simulink model "RR_interaction"  (R2020b)
settings: Solver=FixedStepAuto  StartTime=0.0  StopTime=10.0  FixedStep=0.001  MaxStep=0.05  RelTol=1e-3
values from neighbouring files (symbols this model uses):
  e_max = 0.01    [init.m]
  F_int_max = [5;5]    [init.m]
  F_max = [4;4]    [init.m]
  g = 9.81    [init.m]
  I1 = 1    [init.m]
  I2 = 1    [init.m]
  l1 = 1    [init.m]
  l2 = 1    [init.m]
  m1 = 1    [init.m]
  m2 = 1    [init.m]
  mass = 1    [init.m]
  ts_bound = 0.05    [init.m]
libraries: cstblocks x2, simulink x1
settings Model: Creator=chiara-s  LastModifiedBy=chiara-s

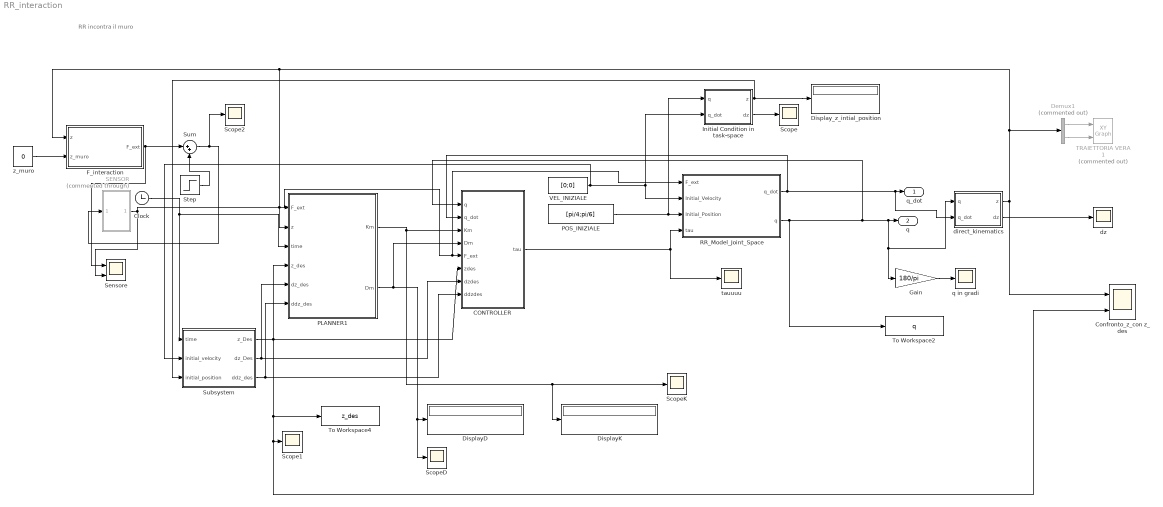
== system RR_interaction ==
  note: RR incontra il muro
  CONTROLLER : MATLAB Function  TreatAsAtomicUnit=on
  Clock : Clock
  Confronto_z_con z_des : Scope  NumInputPorts=2
  Demux1 : Demux  Commented=on  Outputs=2
  DisplayD : Display
  DisplayK : Display
  Display_z_intial_position : Display
  F_interaction : MATLAB Function  TreatAsAtomicUnit=on
  Gain : Gain  Gain=180/pi
  Initial Condition in task-space : MATLAB Function  TreatAsAtomicUnit=on
  PLANNER1 : MATLAB Function  TreatAsAtomicUnit=on
  POS_INIZIALE : Constant  Value=[pi/4;pi/6]
  RR_Model_Joint_Space : Subsystem
  SENSOR : Subsystem  Commented=through
  Scope : Scope
  Scope1 : Scope
  Scope2 : Scope
  ScopeD : Scope
  ScopeK : Scope
  "Sensore " : Scope  NumInputPorts=2
  Step : Step  Time=0  After=[F_max(1);0]  SampleTime=0
  Subsystem : Subsystem
  Sum : Sum  Inputs=|++
  TRAIETTORIA VERA 1 : simulink/Sinks/XY Graph  Commented=on  xmin=-2  xmax=2  ymin=-2  ymax=2  st=-1
  To Workspace2 : ToWorkspace  VariableName=q  SaveFormat=Structure With Time  SampleTime=-1
      settings: Save2DSignal=2-D array (concatenate along first dimension)
  To Workspace4 : ToWorkspace  VariableName=z_des  SaveFormat=Structure With Time  SampleTime=-1
      settings: Save2DSignal=2-D array (concatenate along first dimension)
  VEL_INIZIALE : Constant  Value=[0;0]
  direct_kinematics : MATLAB Function  TreatAsAtomicUnit=on
  dz : Scope
  q in gradi : Scope
  tauuuu : Scope
  z_muro : Constant  Value=0
  q_dot : Outport
  q : Outport  Port=2
  wires:
  z_muro/1 -> F_interaction/2(z_muro)
  direct_kinematics/1(z) -> Confronto_z_con z_des/1, PLANNER1/2(z), F_interaction/1(z), Demux1/1
  Clock/1 -> Subsystem/1(time), PLANNER1/3(time)
  Demux1/2 -> TRAIETTORIA VERA 1/2
  Subsystem/2(dz_Des) -> PLANNER1/5(dz_des), CONTROLLER/7(dzdes)
  VEL_INIZIALE/1 -> Subsystem/2(initial_velocity), Initial Condition in task-space/2(q_dot), RR_Model_Joint_Space/2(Initial_Velocity)
  CONTROLLER/1(tau) -> tauuuu/1, RR_Model_Joint_Space/4(tau)
  Initial Condition in task-space/2(dz) -> Scope/1
  direct_kinematics/2(dz) -> dz/1
  Subsystem/1(z_Des) -> PLANNER1/4(z_des), CONTROLLER/6(zdes), Confronto_z_con z_des/2, Scope1/1, To Workspace4/1
  POS_INIZIALE/1 -> RR_Model_Joint_Space/3(Initial_Position), Initial Condition in task-space/1(q)
  RR_Model_Joint_Space/2(q) -> CONTROLLER/1(q), Gain/1, direct_kinematics/1(q), q/1, To Workspace2/1
  Subsystem/3(ddz_des) -> PLANNER1/6(ddz_des), CONTROLLER/8(ddzdes)
  SENSOR/1(F_ext) -> RR_Model_Joint_Space/1(F_ext), CONTROLLER/5(F_ext), PLANNER1/1(F_ext), "Sensore "/2
  Gain/1 -> q in gradi/1
  Initial Condition in task-space/1(z) -> Subsystem/3(initial_position), Display_z_intial_position/1
  RR_Model_Joint_Space/1(q_dot) -> direct_kinematics/2(q_dot), q_dot/1, CONTROLLER/2(q_dot)
  Demux1/1 -> TRAIETTORIA VERA 1/1
  PLANNER1/1(Km) -> DisplayK/1, ScopeK/1, CONTROLLER/3(Km)
  PLANNER1/2(Dm) -> CONTROLLER/4(Dm), ScopeD/1, DisplayD/1
  F_interaction/1(F_ext) -> "Sensore "/1, Sum/1
  Sum/1 -> Scope2/1, SENSOR/1(In1)
  Step/1 -> Sum/2

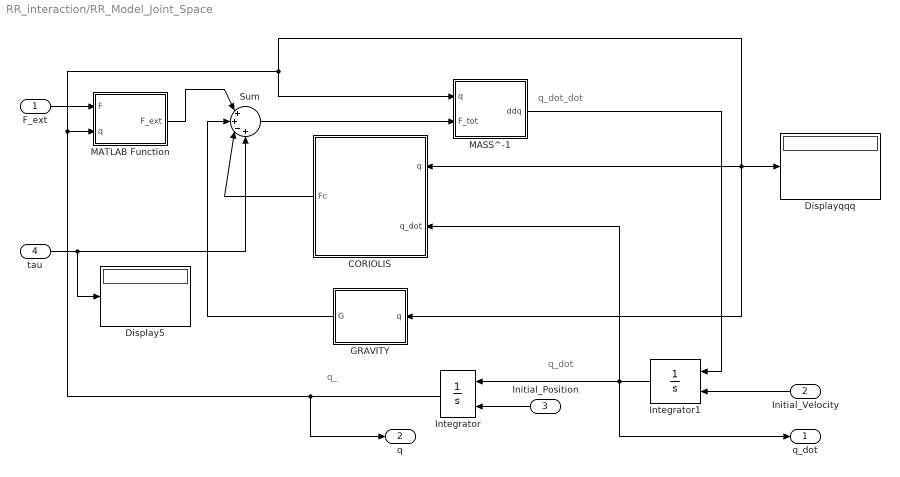
== system RR_interaction/RR_Model_Joint_Space ==
  note: q_dot
  note: q_dot_dot
  note: q_
  F_ext : Inport
  Initial_Velocity : Inport  Port=2
  Initial_Position : Inport  Port=3
  tau : Inport  Port=4
  CORIOLIS : MATLAB Function  TreatAsAtomicUnit=on
  Display5 : Display
  Displayqqq : Display
  GRAVITY : MATLAB Function  TreatAsAtomicUnit=on
  Integrator : Integrator  InitialConditionSource=external
  Integrator1 : Integrator  InitialConditionSource=external  InitialCondition=[0;0]
  MASS^-1 : MATLAB Function  TreatAsAtomicUnit=on
  MATLAB Function : MATLAB Function  TreatAsAtomicUnit=on
  Sum : Sum  Inputs=|++-+
  q_dot : Outport
  q : Outport  Port=2
  wires:
  GRAVITY/1(G) -> Sum/2
  MATLAB Function/1(F_ext) -> Sum/1
  Initial_Position/1 -> Integrator/2
  F_ext/1 -> MATLAB Function/1(F)
  Integrator/1 -> MASS^-1/1(q), GRAVITY/1(q), Displayqqq/1, CORIOLIS/1(q), MATLAB Function/2(q), q/1
  Integrator1/1 -> q_dot/1, CORIOLIS/2(q_dot), Integrator/1
  Initial_Velocity/1 -> Integrator1/2
  MASS^-1/1(ddq) -> Integrator1/1
  Sum/1 -> MASS^-1/2(F_tot)
  CORIOLIS/1(Fc) -> Sum/3
  tau/1 -> Display5/1, Sum/4

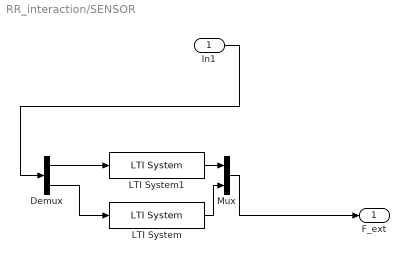
== system RR_interaction/SENSOR ==
  In1 : Inport
  Demux : Demux  Outputs=2
  LTI System : cstblocks/LTI System  sys=tf(200^2,[1 0.5*2*200 200^2])  IC=[]
  LTI System1 : cstblocks/LTI System  sys=tf(200^2,[1 0.5*2*200 200^2])  IC=[]
  Mux : Mux  Inputs=2
  F_ext : Outport
  wires:
  LTI System1/1 -> Mux/1
  Demux/1 -> LTI System1/1
  Demux/2 -> LTI System/1
  LTI System/1 -> Mux/2
  Mux/1 -> F_ext/1
  In1/1 -> Demux/1

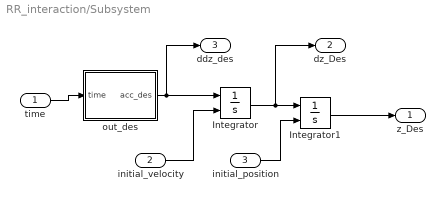
== system RR_interaction/Subsystem ==
  time : Inport
  initial_velocity : Inport  Port=2
  initial_position : Inport  Port=3
  Integrator : Integrator  InitialConditionSource=external
  Integrator1 : Integrator  InitialConditionSource=external
  out_des : MATLAB Function  TreatAsAtomicUnit=on
  z_Des : Outport
  dz_Des : Outport  Port=2
  ddz_des : Outport  Port=3
  wires:
  Integrator1/1 -> z_Des/1
  time/1 -> out_des/1(time)
  Integrator/1 -> dz_Des/1, Integrator1/1
  out_des/1(acc_des) -> ddz_des/1, Integrator/1
  initial_velocity/1 -> Integrator/2
  initial_position/1 -> Integrator1/2

== matlab function RR_interaction/RR_Model_Joint_Space/MASS^-1 ==
  data: q input size=2; ddq output size=2; F_tot input double size=2; I1 parameter; I2 parameter; l1 parameter; l2 parameter; m1 parameter; m2 parameter
function ddq = fcn(q,F_tot,I1, I2, l1, l2, m1, m2)


B = [((l1^2)/4)*m1 + I1 + m2*(l1^2) + m2*((l2^2)/4) + m2*l1*l2*cos(q(2)) + I2, m2*(((l1*l2)/2)*cos(q(2)) + (l2^2)/4) + I2; ...
    m2*(((l1*l2)/2)*cos(q(2)) + (l2^2)/4) + I2, m2*(l2^2)/4 + I2];


ddq = B\F_tot;                      % Ftot*M^-1

end

== matlab function RR_interaction/RR_Model_Joint_Space/MATLAB Function ==
  data: F input size=2; F_ext output double size=2; q input size=2; l1 parameter; l2 parameter
function F_ext = fcn(F,q,l1, l2)


Ja = [-l1*sin(q(1)) - l2*sin(q(1)+q(2)), -l2*sin(q(1)+q(2)); ...
    l1*cos(q(1)) + l2*cos(q(1)+q(2)), l2*cos(q(1)+q(2))];

F_ext = Ja'*F;

end

== matlab function RR_interaction/direct_kinematics ==
  data: q input double size=2; q_dot input double size=2; z output double size=2; dz output double size=2; l1 parameter; l2 parameter
function [z,dz] = fcn(q,q_dot,l1, l2)

z = zeros(2,1);
z(1) = l1*cos(q(1)) + l2*cos(q(1)+q(2));
z(2) = l1*sin(q(1)) + l2*sin(q(1)+q(2));

Ja = zeros(2,2);
Ja = [-l1*sin(q(1)) - l2*sin(q(1)+q(2)), -l2*sin(q(1)+q(2)); ...
    l1*cos(q(1)) + l2*cos(q(1)+q(2)), l2*cos(q(1)+q(2))];

dz = zeros(2,1);
dz = Ja*q_dot;

end

== matlab function RR_interaction/Subsystem/out_des ==
  settings: sampleTime=0.1
  data: time input; acc_des output
function acc_des = fcn(time)
%% desired trajectory generator
if time < 0.1
    acc_des = [-5;0]; 
elseif time < 3.1
    acc_des = [0;0];
elseif time < 3.2
    acc_des = [5;0];
else 
    acc_des = [0;0];
end


end

== matlab function RR_interaction/F_interaction ==
  data: z input; F_ext output; z_muro input
function F_ext = fcn(z, z_muro)
% hypothesis: table reaction force with elastic behaviour
F_ext = zeros(2,1);
K = 100000;         % 1 mm displacement for 10 kg
F_ext(1) = 0;
F_ext(2) = 0;
% if contact is happened
if z_muro > z(1)
    F_ext(1) = K*(z_muro - z(1));
end

== matlab function RR_interaction/PLANNER1 ==
  settings: updateMethod=DISCRETE
  data: F_max parameter; Km output; Dm output; e_max parameter; F_ext input; z input; time input; z_des input; dz_des input; ddz_des input; F_int_max parameter; mass parameter; ts_bound parameter
function [Km,Dm] = fcn(F_max, e_max,F_ext, z,time, z_des, dz_des, ddz_des, F_int_max, mass, ts_bound)

%% Description MDS_interaction
% decrease k after contact is sensed to limit the interaction force

%% Outputs
% Km            stiffness matrix
% Dm            damping matrix

%% Inputs
% time          current simulation time
% F_ext         measured external force
% mass          mass scalar value 
% F_int_max     desired interaction force
% z_des, dz_des, ddz_des                    desired trajectory
% z             current position
% F_max         estimated force disturbances
% e_max         maximum steady-state error

persistent F_prec kx ky dx dy t_changex t_changey t_settlx t_settly t_interaction

% time of a first interaction
if isempty(t_interaction)
    t_interaction = 1000;
end

% settling time
if isempty(t_settlx)
    t_settlx = 0;
end
if isempty(t_settly)
    t_settly = 0;
end

% time of last stiffness update
if isempty(t_changex)
    t_changex = 1000;
end
if isempty(t_changey)
    t_changey = 1000;
end

% previous measured force
if isempty(F_prec)
    F_prec = [0;0];
end

% initialization of k and d 
if isempty(kx)
   kx = F_max(1)/e_max; 
end
if isempty(ky)
   ky = F_max(2)/e_max;
end
if isempty(dx)
    dx = sqrt(4*kx*mass);
end
if isempty(dy)
    dy = sqrt(4*ky*mass);
end


if abs(F_ext(1)) > F_int_max(1) 
    % set t_interaction once contact is sensed
    if t_interaction == 1000
        t_interaction = time;
    end
    % if force is increasing
    if abs(F_prec(1)) < abs(F_ext(1))
        % if interaction force is higher than threshold
        if kx*abs(z(1)-z_des(1)) > F_int_max(1)
            % set k 
            kx = F_int_max(1)/abs(z(1)-z_des(1));
            % kx = 0.98*kx;
            dx = sqrt(4*kx*mass);

        end
    end
end
% Similarly for the other direction
if abs(F_ext(2)) > F_int_max(2) 
    if t_interaction == 1000
       t_interaction = time;
    end
    if abs(F_prec(2)) < abs(F_ext(2))
        if ky*abs(z(2)-z_des(2)) > F_int_max(2)
            ky = F_int_max(2)/abs(z(2)-z_des(2));
            % ky = 0.98*ky;
            dy = sqrt(4*ky*mass);
        end
    end
end

F_prec = F_ext;     % update for last force

% set final values 
Dm = diag([dx,dy]);
Km = diag([kx,ky]);
end

== matlab function RR_interaction/CONTROLLER ==
  data: q input size=2; q_dot input size=2; Km input; Dm input; F_ext input; M parameter; zdes input size=2; tau output double size=2; dzdes input size=2; ddzdes input size=2
function tau = fcn(q, q_dot, Km, Dm, F_ext, M, zdes, dzdes, ddzdes)

coder.extrinsic('Jacobianoa','Jacobianoa_dot','Mass','Coriolis','Gravity','cin_dir')
dz = zeros(2,1);
z = zeros(2,1);
B = zeros(2,2);
S = zeros(2,2);
G = zeros(2,1);
Ja = zeros(2,2);
Ja_dot = zeros(2,2);
Bm = [M 0; 0 M];
Ja = Jacobianoa(q);
Ja_dot = Jacobianoa_dot(q,q_dot);

dz = Ja*q_dot;
z = cin_dir(q);

t = 0.1;
if (deg2rad(-0.1) < q(2)) && (q(2) < deg2rad(0.1)) || (deg2rad(179.9) < q(2)) && (q(2) < deg2rad(180.1)) || (deg2rad(-180.1) < q(2)) && (q(2) < deg2rad(-179.9))
    Ja_inv = (Ja')*inv(Ja*(Ja') + t^2*eye(2,2)); % Damp least square Jacobian method
else 
    Ja_inv = inv(Ja);
end

% Ja_inv = inv(Ja);

B = Mass(q);
Bx = (Ja_inv')* B * Ja_inv;
S = Coriolis(q,q_dot);
G = Gravity(q);
I = eye(2,2);
% tau = B * Ja_inv*(ddzdes - Ja_dot*q_dot) + ...
%     S*q_dot + (Ja')*(Dm*(dzdes - dz) + Km*(zdes- z)) + G;

tau = B*Ja_inv*(ddzdes - Ja_dot*q_dot + ...
    inv(Bm)*(Dm*(dzdes - dz) + Km*(zdes- z))) + S*q_dot - G + ...
    (Ja')*(Bx*inv(Bm) - I)*F_ext;

end

== matlab function RR_interaction/Initial Condition in task-space ==
  data: q input double size=2; q_dot input double size=2; z output double size=2; dz output double size=2; l1 parameter; l2 parameter
function [z,dz] = fcn(q,q_dot,l1, l2)

z = zeros(2,1);
z(1) = l1*cos(q(1)) + l2*cos(q(1)+q(2));
z(2) = l1*sin(q(1)) + l2*sin(q(1)+q(2));

Ja = zeros(2,2);
Ja = [-l1*sin(q(1)) - l2*sin(q(1)+q(2)), -l2*sin(q(1)+q(2)); ...
    l1*cos(q(1)) + l2*cos(q(1)+q(2)), l2*cos(q(1)+q(2))];

dz = zeros(2,1);
dz = Ja*q_dot;

end

== matlab function RR_interaction/RR_Model_Joint_Space/CORIOLIS ==
  data: q input size=2; Fc output double size=2; q_dot input size=2; a parameter
function Fc = fcn(q,q_dot,a)

C = zeros(2,2);
C = [-a*sin(q(2))*q_dot(2), -a*sin(q(2))*q_dot(1)-a*sin(q(2)*q_dot(2)); ...
    a*sin(q(2))*q_dot(1), 0];

Fc = C*q_dot;

end

== matlab function RR_interaction/RR_Model_Joint_Space/GRAVITY ==
  data: q input size=2; G output double size=2; g parameter; l1 parameter; l2 parameter; m1 parameter; m2 parameter
function G = fcn(q,g, l1, l2, m1, m2)


G = [-(l1/2)*cos(q(1))*m1*g - m2*g*(l1*cos(q(1))+(l2/2)*cos(q(1)+q(2))); ...
    -m2*g*(l2/2)*cos(q(1)+q(2))];

end
